simulink model "Controlador_P_de_Corrientes"  (R2023b)
settings: Solver=VariableStepAuto  StartTime=0.0  StopTime=10.0  RelTol=1e-3
values from neighbouring files (symbols this model uses):
  L_d = 6.6e-3    (= 0.0066)    [controlador_foc_simulink.m]    (also in params_subsistema_electromagnetico.m; sistema_completo_en_codigo.m)
  L_l = 0.8e-3    (= 0.0008)    [controlador_foc_simulink.m]    (also in params_subsistema_electromagnetico.m; sistema_completo_en_codigo.m)
  L_q = 5.8e-3    (= 0.0058)    [controlador_foc_simulink.m]    (also in params_subsistema_electromagnetico.m; sistema_completo_en_codigo.m)
settings Model: Creator=Pc  LastModifiedBy=Pc

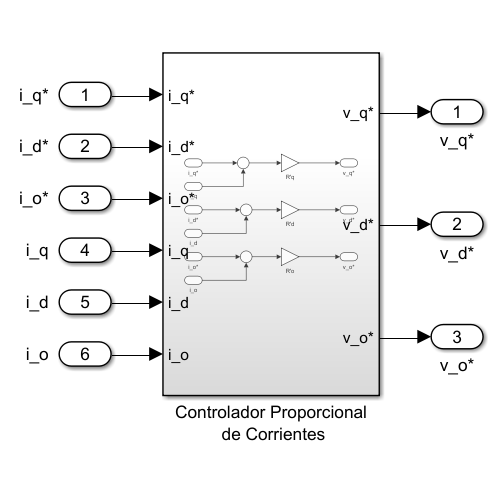
[thumbnail: Simulink's stored preview of the top-level diagram]
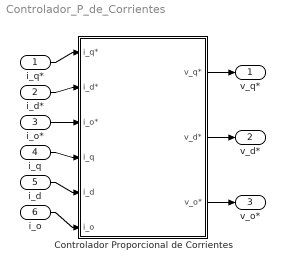
== system Controlador_P_de_Corrientes ==
  i_q* : Inport
  i_d* : Inport  Port=2
  i_o* : Inport  Port=3
  i_q : Inport  Port=4
  i_d : Inport  Port=5
  i_o : Inport  Port=6
  Controlador Proporcional de Corrientes : Subsystem
  v_q* : Outport
  v_d* : Outport  Port=2
  v_o* : Outport  Port=3
  wires:
  i_q*/1 -> Controlador Proporcional de Corrientes/1(i_q*)
  i_d*/1 -> Controlador Proporcional de Corrientes/2(i_d*)
  i_o*/1 -> Controlador Proporcional de Corrientes/3(i_o*)
  i_q/1 -> Controlador Proporcional de Corrientes/4(i_q)
  i_d/1 -> Controlador Proporcional de Corrientes/5(i_d)
  i_o/1 -> Controlador Proporcional de Corrientes/6(i_o)
  Controlador Proporcional de Corrientes/1(v_q*) -> v_q*/1
  Controlador Proporcional de Corrientes/2(v_d*) -> v_d*/1
  Controlador Proporcional de Corrientes/3(v_o*) -> v_o*/1

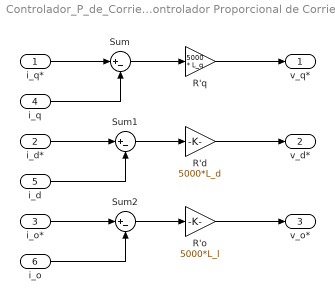
== system Controlador_P_de_Corrientes/Controlador Proporcional de Corrientes ==
  i_q* : Inport
  i_d* : Inport  Port=2
  i_o* : Inport  Port=3
  i_q : Inport  Port=4
  i_d : Inport  Port=5
  i_o : Inport  Port=6
  R'd : Gain  Gain=5000*L_d
  R'o : Gain  Gain=5000*L_l
  R'q : Gain  Gain=5000 * L_q
  Sum : Sum  Inputs=|+-
  Sum1 : Sum  Inputs=|+-
  Sum2 : Sum  Inputs=|+-
  v_q* : Outport
  v_d* : Outport  Port=2
  v_o* : Outport  Port=3
  wires:
  R'd/1 -> v_d*/1
  i_q/1 -> Sum/2
  i_d*/1 -> Sum1/1
  R'o/1 -> v_o*/1
  i_o*/1 -> Sum2/1
  Sum/1 -> R'q/1
  Sum1/1 -> R'd/1
  i_o/1 -> Sum2/2
  Sum2/1 -> R'o/1
  R'q/1 -> v_q*/1
  i_d/1 -> Sum1/2
  i_q*/1 -> Sum/1
